simulink model "xmc_fir_import"  (R2019b)
settings: Solver=VariableStepAuto  StartTime=0.0  StopTime=inf  RelTol=1e-3
PostLoadFcn:
  | xmcHubUpdateInstalledDevice(gcs);
undefined symbols (not defined in the file or in its folder): xc7vx485tffg1157
libraries: ModelComposer x3, xmcCopyrightNotice x1, dspsrcs4 x1, fir_c_import x1
settings Model: Creator=abehbood  LastModifiedBy=abehbood
settings DataIOCC: ReturnWorkspaceOutputs=off
settings OptimizationCC: LifeSpan=inf
settings DebuggingCC: ArithmeticOperatorsInVariantConditions=warning
settings SFSimCC: SimUseLocalCustomCode=off  CustomCodeUndefinedFunction=UseInterfaceOnly
settings RTWCC: RTWUseLocalCustomCode=off
settings CodeAppCC: StateflowObjectComments=on

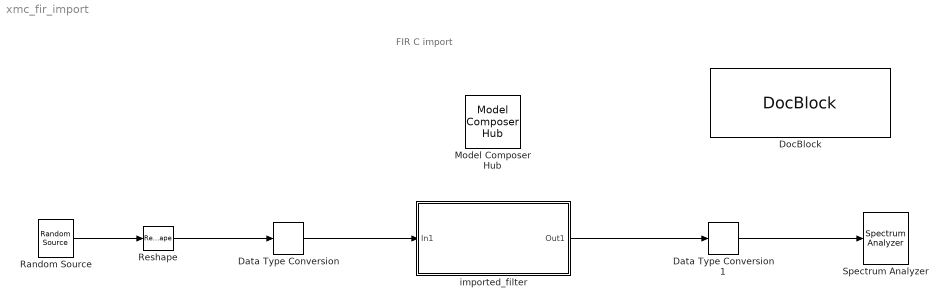
== system xmc_fir_import ==
  note: FIR C import
  Data Type Conversion : ModelComposer/Data Type Conversion  OutDataType=fixed  TypeExp=''  Signedness=Signed  WordLength=17  FractionalLength=14  RoundingMode=Truncation to minus infinity  OverflowMode=Wrap around
  Data Type Conversion1 : ModelComposer/Data Type Conversion  OutDataType=double  TypeExp=''  Signedness=Signed  WordLength=16  FractionalLength=0  RoundingMode=Truncation to minus infinity  OverflowMode=Wrap around
  DocBlock : xmcCopyrightNotice/DocBlock
      content=|
      | (c) Copyright 2017-2018 Xilinx, Inc. All rights reserved.
      |
      | This file contains confidential and proprietary information of Xilinx, Inc.
      | and is protected under U.S. and international copyright and other
      | intellectual property laws.
      |
      | DISCLAIMER
      | This disclaimer is not a license and does not grant any rights to the
      | materials distributed herewith. Except as otherwise provided in a valid
      | license issued to you by Xilinx, and to the maximum extent permitted by
      | applicable law: (1) THESE MATERIALS ARE MADE AVAILABLE "AS IS" AND WITH
      | ALL FAULTS, AND XILINX HEREBY DISCLAIMS ALL WARRANTIES AND CONDITIONS,
      | EXPRESS, IMPLIED, OR STATUTORY, INCLUDING BUT NOT LIMITED TO WARRANTIES
      | OF MERCHANTABILITY, NON-INFRINGEMENT, OR FITNESS FOR ANY PARTICULAR
      | PURPOSE; and (2) Xilinx shall not be liable (whether in contract or tort,
      | including negligence, or under any other theory of liability) for any
      | loss or damage of any kind or nature related to, arising under or in
      | connection with these materials, including for any direct, or any indirect,
      | special, incidental, or consequential loss or damage (including loss of
      | data, profits, goodwill, or any type of loss or damage suffered as a
      | result of any action brought by a third party) even if such damage or loss
      | was reasonably foreseeable or Xilinx had been advised of the possibility
      | of the same.
      |
      | CRITICAL APPLICATIONS
      | Xilinx products are not designed or intended to be fail-safe, or for use
      | in any application requiring fail-safe performance, such as life-support
      | or safety devices or systems, Class III medical devices, nuclear
      | facilities, applications related to the deployment of airbags, or
      | any other applications that could lead to death, personal injury, or
      | severe property or environmental damage (individually and collectively,
      | "Critical Applications"). Customer assumes the sole risk and liability
      | of any use of Xilinx products in Critical Applications, subject only to
      | applicable laws and regulations governing limitations on product liability.
      |
      | THIS COPYRIGHT NOTICE AND DISCLAIMER MUST BE RETAINED AS PART OF
      | THIS FILE AT ALL TIMES.
      settings: SourceProductName=Simulink  SourceProductBaseCode=SL
  Model Composer Hub : ModelComposer/Model Composer Hub  CodeGeneration=off  SubsystemName=imported_filter  TargetDirectory=./code  ExportType=HLS C++ code  IpVendor=xilinx.com  IpLibrary=hls  IpVersion=1.0  IpHWLanguage=Verilog  AieCompilerOptions={}  CreateTestbench=off  TestbenchStackSize=10  RunAieSim=off  AieSimTimeout=50000  LaunchVitisAnalyzer=off  RunX86Sim=on  X86SimTimeout=10  ProjDevice=xc7vx485tffg1157-1  ProjDevicePart=xc7vx485tffg1157-1  SamplePeriod=-1  ClockFrequency=200  DataPathParallelism=1
  Random Source : dspsrcs4/Random Source  SrcType=Gaussian  NormMethod=Ziggurat  CltLength=12  MinVal=0  MaxVal=1  MeanVal=0  VarVal=1  RepMode=Not repeatable  rawSeed=1  IsInherit=off  SampMode=Discrete  SampTime=1  SampFrame=100  DataType=Double  OutComplex=Real  OutputFrames=off
  Reshape : Reshape
  Spectrum Analyzer : SpectrumAnalyzer
  imported_filter : Subsystem
  wires:
  Data Type Conversion1/1 -> Spectrum Analyzer/1
  Random Source/1 -> Reshape/1
  Data Type Conversion/1 -> imported_filter/1(In1)
  imported_filter/1(Out1) -> Data Type Conversion1/1
  Reshape/1 -> Data Type Conversion/1

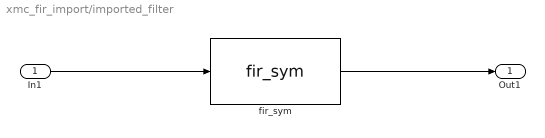
== system xmc_fir_import/imported_filter ==
  In1 : Inport
  fir_sym : fir_c_import/fir_sym  LibraryFunction=fir_sym  IncludeFiles={'fir_sym.h'}  SourceFiles={'fir.h', 'fir_sym.cpp', 'coef_halfof103.inc'}  IncludeDirectories={}  TemplateParams={' '}  FunctionParamTypes={xmcDataType('void'); xmcDataType('ap_fixed<17, 3, AP_TRN, AP_WRAP>'); xmcDataType('ap_fixed<17, 3, AP_TRN, AP_WRAP>')}  FunctionParamPassbys={0.000000000000000000e+00; 0.000000000000000000e+00; 0.000000000000000000e+00}  FunctionParamDimensions={'1'; '[100]'; '[100]'}  FunctionParamNames={'return'; 'din'; 'dout'}  FunctionParamDir={0.000000000000000000e+00; 1.000000000000000000e+00; 2.000000000000000000e+00}  FunctionParamSupportsStreaming={true; true; true}  BufferDepth={'0'}  FunctionParamValues={'0'; '0'; '0'}  ThroughputFactors={''}
  Out1 : Outport
  wires:
  In1/1 -> fir_sym/1
  fir_sym/1 -> Out1/1
